simulink model "M_ZH_Z5"  (R2025a)
settings: Solver=ode45  StartTime=0.0  StopTime=10e-3  MaxStep=25e-6/25  RelTol=1e-3  EnableMultiTasking=on
libraries: M_MK x1
settings Model: Creator=oktato  LastModifiedBy=Szalay
settings SolverCC: AlgebraicLoopSolver=TrustRegion
settings DataIOCC: LimitDataPoints=on  SaveFormat=Array  ReturnWorkspaceOutputs=off
settings OptimizationCC: LifeSpan=inf
settings DebuggingCC: UnderspecifiedInitializationDetection=Classic  MergeDetectMultiDrivingBlocksExec=none  SolverPrmCheckMsg=warning  UnconnectedInputMsg=warning  UnconnectedOutputMsg=warning  UnconnectedLineMsg=warning  SFUnexpectedBacktrackingDiag=warning  SFNoUnconditionalDefaultTransitionDiag=warning  SFExecutionAtInitializationDiag=none  ArithmeticOperatorsInVariantConditions=warning
settings HardwareCC: ProdBitPerPointer=32.0  ProdBitPerSizeT=32.0  ProdBitPerPtrDiffT=32.0  ProdLargestAtomicFloat=None  ProdIntDivRoundTo=Undefined  ProdEndianess=Unspecified  ProdWordSize=32.0  ProdHWDeviceType=32-bit Generic
settings ModelReferenceCC: PropagateSignalLabelsOutOfModel=off
settings SFSimCC: SimUseLocalCustomCode=off  CustomCodeUndefinedFunction=UseInterfaceOnly
settings RTWCC: RTWUseLocalCustomCode=off  GPUComputeCapability=3.5
settings CodeAppCC: StateflowObjectComments=on
settings GRTTargetCC: TargetLangStandard=C89/C90 (ANSI)
settings ConfigComp: CovMetricSettings=dw  CovSaveCumulativeToWorkspaceVar=on  CovSaveSingleToWorkspaceVar=on  CovExternalEMLEnable=off

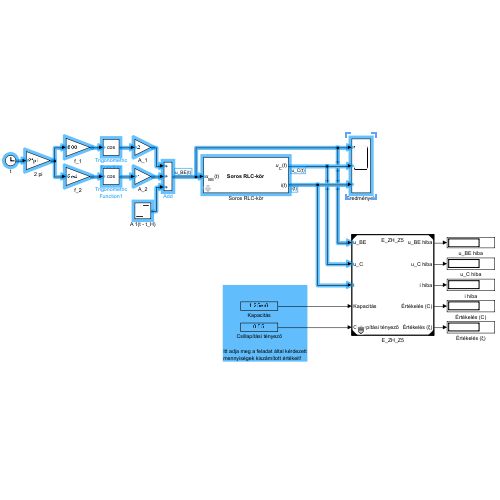
[thumbnail: Simulink's stored preview of the top-level diagram]
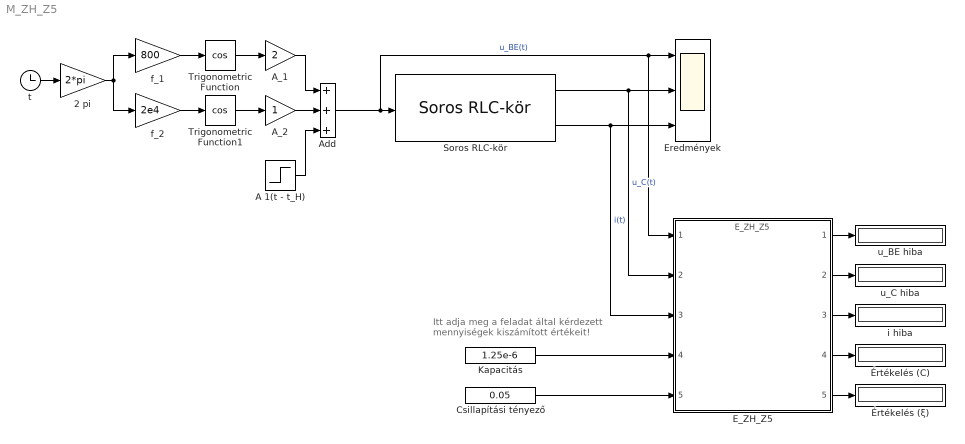
== system M_ZH_Z5 ==
  note: Itt adja meg a feladat által kérdezett
      | mennyiségek kiszámított értékeit!
  2 pi : Gain  Gain=2*pi
  A 1(t - t_H) : Step  Time=5e-3  After=5  SampleTime=0
  A_1 : Gain  Gain=2
  A_2 : Gain
  Add : Sum  Inputs=+++
  Csillapítási tényező : Constant  Value=0.05
  E_ZH_Z5 : ModelReference  ModelNameDialog=E_ZH_Z5.slxp  ModelReferenceVersion=1.13  CopyOfModelProtected=on
  Eredmények : Scope  NumInputPorts=3
      settings: ActiveDisplayYMinimum=-4.375  ActiveDisplayYMaximum=9.375
  Kapacitás : Constant  Value=1.25e-6
  Soros RLC-kör : M_MK/Soros RLC-kör  L=500e-6  R=2  tau=25e-6  u_C0=1  i_0=-200e-3
  Trigonometric Function : Trigonometry  Operator=cos
  Trigonometric Function1 : Trigonometry  Operator=cos
  f_1 : Gain  Gain=800
  f_2 : Gain  Gain=2e4
  i hiba : Display
  t : Clock
  u_BE hiba : Display
  u_C hiba : Display
  Értékelés (C) : Display
  Értékelés (ξ) : Display
  wires:
  t/1 -> 2 pi/1
  f_1/1 -> Trigonometric Function/1
  Trigonometric Function/1 -> A_1/1
  A_1/1 -> Add/1
  A 1(t - t_H)/1 -> Add/3
  Add/1 -> Soros RLC-kör/1, E_ZH_Z5/1, Eredmények/1  "u_BE(t)"
  Soros RLC-kör/1 -> E_ZH_Z5/2, Eredmények/2  "u_C(t)"
  Soros RLC-kör/2 -> E_ZH_Z5/3, Eredmények/3  "i(t)"
  Trigonometric Function1/1 -> A_2/1
  f_2/1 -> Trigonometric Function1/1
  A_2/1 -> Add/2
  2 pi/1 -> f_1/1, f_2/1
  E_ZH_Z5/3 -> i hiba/1
  E_ZH_Z5/1 -> u_BE hiba/1
  E_ZH_Z5/2 -> u_C hiba/1
  Kapacitás/1 -> E_ZH_Z5/4
  Csillapítási tényező/1 -> E_ZH_Z5/5
  E_ZH_Z5/5 -> Értékelés (ξ)/1
  E_ZH_Z5/4 -> Értékelés (C)/1
